simulink model "ProjectFinal"  (R2019a)
settings: Solver=ode45  StartTime=0.6  StopTime=1  MaxStep=1e-7  MinStep=1e-8  RelTol=1e-3
undefined symbols (not defined in the file): sigbuilder_block
libraries: powerlib x55, simulink x10, dspstat3 x2, re_lib x1
(part 1 of 2)
settings Model: Creator=Nabila Tasnim  LastModifiedBy=Nabila Tasnim

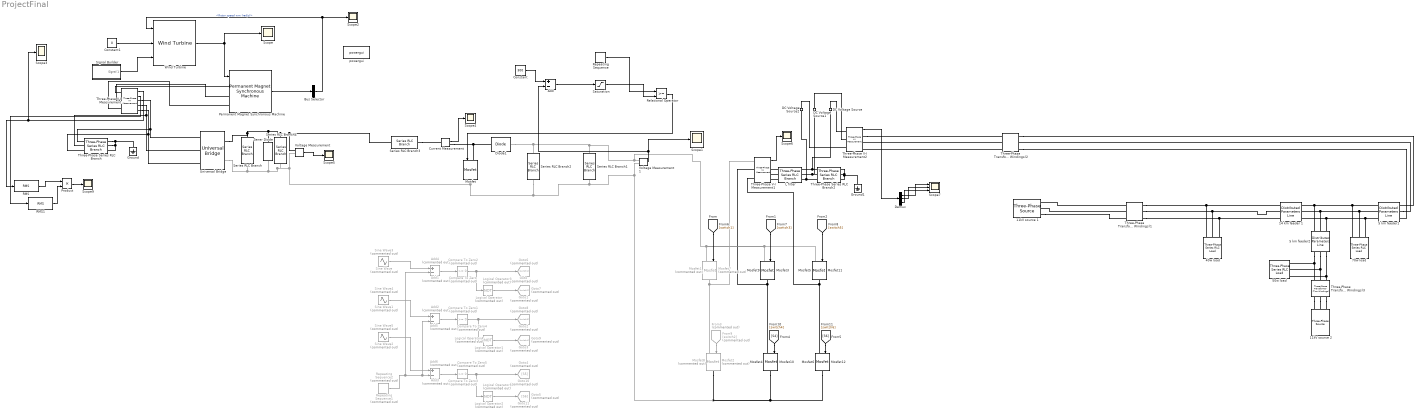
== system ProjectFinal ==
  11kV source 1 : powerlib/Electrical Sources/Three-Phase Source  InternalConnection=Yg  VoltagePhases=off  Voltage=11e3*(1/sqrt(2))  PhaseAngle=0  Voltage_phases=[25e3 25e3 25e3]/sqrt(3)  PhaseAngles_phases=[0 -120 +120]  Frequency=60  NonIdealSource=on  SpecifyImpedance=off  Resistance=0.8929  Inductance=0  ShortCircuitLevel=100e6  BaseVoltage=25e3  XRratio=7  BusType=swing  Pref=0  Qref=0  Prefabc=[10e3, 10e3, 10e3]  Qrefabc=[0, 0, 0]  Qmin=-inf  Qmax=inf
      settings: SourceProductName=Simscape Electrical
  11kV source 2 : powerlib/Electrical Sources/Three-Phase Source  InternalConnection=Yg  VoltagePhases=off  Voltage=11e3*(1/sqrt(2))  PhaseAngle=0  Voltage_phases=[25e3 25e3 25e3]/sqrt(3)  PhaseAngles_phases=[0 -120 +120]  Frequency=60  NonIdealSource=on  SpecifyImpedance=off  Resistance=0.8929  Inductance=0  ShortCircuitLevel=100e6  BaseVoltage=25e3  XRratio=7  BusType=swing  Pref=0  Qref=0  Prefabc=[10e3, 10e3, 10e3]  Qrefabc=[0, 0, 0]  Qmin=-inf  Qmax=inf
      settings: SourceProductName=Simscape Electrical
  14 km feeder 1 : powerlib/Elements/Distributed Parameters Line  Phases=3  Frequency=50  Resistance=[0.01273 0.003864]  Inductance=[0.001 0.001]  Capacitance=[0.001 0.001]  Length=10  x1=[-0.01 -3.68951467134757e-09 40.0386247368383 386.049187884333;-0.0099995 -3.68951467134757e-09 39.9658554684164 386.056728128973;-0.009999 -3.68951467134757e-09 39.8930847799852 386.064254656796;-0.0099985 -3.68951467134757e-09 39.8203126741293 386.071767467533;-0.009998 -3.68951467134757e-09 39.7475391534347 386.079266560918;-0.0099975 -3.68951467134757e-09 39.6747642204872 386.086751936685;-0.009997 -3.68951467134757e-09 39.6019878778729 386.094223594567;-0.0099965 -3.68951467134757e-09 39.5292101281768 386.101681534299;-0.009996 -3.68951467134757e-09 39.456430973985 386.109125755615;-0.0099955 -3.68951467134757e-09 39.3836504178839 386.116556258253;-0.009995 -3.68951467134757e-09 39.3108684624588 386.123973041946;-0.0099945 -3.68951467134757e-09 39.2380851102958 386.131376106433;-0.009994 -3.68951467134757e-09 39.1653003639809 386.13876545145;-0.0099935 -3.68951467134757e-09 39.0925142261009 386.146141076733;-0.009993 -3.68951467134757e-09 39.019726699241 386.153502982023;-0.0099925 -3.68951467134757e-09 38.9469377859875 386.160851167056;-0.009992 -3.68951467134757e-09 38.8741474889275 386.168185631571;-0.0099915 -3.68951467134757e-09 38.8013558106463 386.175506375309;-0.009991 -3.68951467134757e-09 38.7285627537305 386.182813398008;-0.0099905 -3.68951467134757e-09 38.6557683207665 386.19010669941;-0.00999 -3.68951467134757e-09 38.5829725143412 386.197386279255;-0.0099895 -3.68951467134757e-09 38.5101753370404 386.204652137284;-0.009989 -3.68951467134757e-09 38.4373767914507 386.21190427324;-0.0099885 -3.68951467134757e-09 38.3645768801595 386.219142686865;-0.009988 -3.68951467134757e-09 38.2917756057523 386.226367377901;-0.0099875 -3.68951467134757e-09 38.2189729708163 386.233578346092;-0.009987 -3.68951467134757e-09 38.1461689779381 386.240775591181;-0.0099865 -3.68951467134757e-09 38.073363629705 386.247959112913;-0.009986 -3.68951467134757e-09 38.000556928703 386.255128911033;-0.0099855 -3.68951467134757e-09 37.9277488775194 386.262284985286;-0.009985 -3.68951467134757e-09 37.8549394787412 386.269427335417;-0.0099845 -3.68951467134757e-09 37.782128734955 386.276555961174;-0.009984 -3.68951467134757e-09 37.709316648748 386.283670862302;-0.0099835 -3.68951467134757e-09 37.6365032227075 386.290772038548;-0.009983 -3.68951467134757e-09 37.5636884594201 386.297859489661;-0.0099825 -3.68951467134757e-09 37.4908723614733 386.304933215389;-0.009982 -3.68951467134757e-09 37.4180549314543 386.31199321548;-0.0099815 -3.68951467134757e-09 37.3452361719503 386.319039489684;-0.009981 -3.68951467134757e-09 37.2724160855485 386.326072037749;-0.0099805 -3.68951467134757e-09 37.1995946748362 386.333090859427;-0.00998 -3.68951467134757e-09 37.1267719424011 386.340095954468;-0.0099795 -3.68951467134757e-09 37.0539478908302 386.347087322622;-0.009979 -3.68951467134757e-09 36.9811225227113 386.354064963643;-0.0099785 -3.68951467134757e-09 36.9082958406317 386.361028877281;-0.009978 -3.68951467134757e-09 36.8354678471794 386.367979063289;-0.0099775 -3.68951467134757e-09 36.7626385449414 386.37491552142;-0.009977 -3.68951467134757e-09 36.6898079365058 386.381838251428;-0.0099765 -3.68951467134757e-09 36.6169760244603 386.388747253067;-0.009976 -3.68951467134757e-09 36.5441428113925 386.395642526091;-0.0099755 -3.68951467134757e-09 36.4713082998902 386.402524070256;-0.009975 -3.68951467134757e-09 36.3984724925412 386.409391885317;-0.0099745 -3.68951467134757e-09 36.3256353919339 386.416245971029;-0.009974 -3.68951467134757e-09 36.2527970006556 386.42308632715;-0.0099735 -3.68951467134757e-09 36.1799573212945 386.429912953436;-0.009973 -3.68951467134757e-09 36.1071163564389 386.436725849644;-0.0099725 -3.68951467134757e-09 36.0342741086765 386.443525015533;-0.009972 -3.68951467134757e-09 35.9614305805956 386.450310450862;-0.0099715 -3.68951467134757e-09 35.8885857747843 386.457082155388;-0.009971 -3.68951467134757e-09 35.8157396938311 386.463840128872;-0.0099705 -3.68951467134757e-09 35.7428923403239 386.470584371073;-0.00997 ...(+1348205 chars)]  x2=[-0.01 -6.7554586962748e-08 -198.081584719035 -137.663501550197;-0.0099995 -6.75545869719076e-08 -198.055632241504 -137.700836603426;-0.009999 -6.75545869810679e-08 -198.029672726942 -137.738166764065;-0.0099985 -6.75545869902288e-08 -198.003706176272 -137.775492030788;-0.009998 -6.75545869993904e-08 -197.977732590417 -137.812812402268;-0.0099975 -6.75545870085525e-08 -197.951751970298 -137.85012787718;-0.009997 -6.75545870177153e-08 -197.92576431684 -137.887438454197;-0.0099965 -6.75545870268788e-08 -197.899769630966 -137.924744131994;-0.009996 -6.75545870360428e-08 -197.873767913599 -137.962044909245;-0.0099955 -6.75545870452075e-08 -197.847759165662 -137.999340784626;-0.009995 -6.75545870543728e-08 -197.821743388082 -138.036631756811;-0.0099945 -6.75545870635388e-08 -197.79572058178 -138.073917824474;-0.009994 -6.75545870727053e-08 -197.769690747683 -138.111198986292;-0.0099935 -6.75545870818725e-08 -197.743653886715 -138.148475240939;-0.009993 -6.75545870910404e-08 -197.717609999801 -138.185746587092;-0.0099925 -6.75545871002088e-08 -197.691559087866 -138.223013023425;-0.009992 -6.75545871093779e-08 -197.665501151837 -138.260274548615;-0.0099915 -6.75545871185476e-08 -197.639436192638 -138.297531161338;-0.009991 -6.75545871277179e-08 -197.613364211197 -138.33478286027;-0.0099905 -6.75545871368888e-08 -197.587285208439 -138.372029644088;-0.00999 -6.75545871460604e-08 -197.561199185291 -138.409271511468;-0.0099895 -6.75545871552326e-08 -197.535106142679 -138.446508461086;-0.009989 -6.75545871644054e-08 -197.509006081532 -138.483740491621;-0.0099885 -6.75545871735788e-08 -197.482899002776 -138.520967601748;-0.009988 -6.75545871827529e-08 -197.456784907339 -138.558189790146;-0.0099875 -6.75545871919276e-08 -197.430663796149 -138.595407055491;-0.009987 -6.75545872011029e-08 -197.404535670133 -138.632619396462;-0.0099865 -6.75545872102788e-08 -197.378400530221 -138.669826811736;-0.009986 -6.75545872194554e-08 -197.352258377341 -138.707029299992;-0.0099855 -6.75545872286325e-08 -197.326109212421 -138.744226859906;-0.009985 -6.75545872378103e-08 -197.299953036391 -138.781419490159;-0.0099845 -6.75545872469887e-08 -197.27378985018 -138.818607189427;-0.009984 -6.75545872561678e-08 -197.247619654717 -138.855789956391;-0.0099835 -6.75545872653474e-08 -197.221442450933 -138.892967789728;-0.009983 -6.75545872745277e-08 -197.195258239758 -138.930140688119;-0.0099825 -6.75545872837086e-08 -197.169067022122 -138.967308650241;-0.009982 -6.75545872928901e-08 -197.142868798955 -139.004471674775;-0.0099815 -6.75545873020722e-08 -197.116663571188 -139.0416297604;-0.009981 -6.7554587311255e-08 -197.090451339753 -139.078782905796;-0.0099805 -6.75545873204383e-08 -197.064232105581 -139.115931109643;-0.00998 -6.75545873296223e-08 -197.038005869603 -139.15307437062;-0.0099795 -6.75545873388069e-08 -197.011772632752 -139.190212687409;-0.009979 -6.75545873479921e-08 -196.985532395959 -139.22734605869;-0.0099785 -6.7554587357178e-08 -196.959285160156 -139.264474483142;-0.009978 -6.75545873663644e-08 -196.933030926276 -139.301597959448;-0.0099775 -6.75545873755515e-08 -196.906769695253 -139.338716486287;-0.009977 -6.75545873847392e-08 -196.880501468019 -139.375830062342;-0.0099765 -6.75545873939275e-08 -196.854226245507 -139.412938686293;-0.009976 -6.75545874031164e-08 -196.827944028651 -139.450042356823;-0.0099755 -6.75545874123059e-08 -196.801654818385 -139.487141072612;-0.009975 -6.7554587421496e-08 -196.775358615642 -139.524234832342;-0.0099745 -6.75545874306868e-08 -196.749055421358 -139.561323634697;-0.009974 -6.75545874398782e-08 -196.722745236467 -139.598407478357;-0.0099735 -6.75545874490701e-08 -196.696428061904 -139.635486362005;-0.009973 -6.75545874582627e-08 -196.670103898603 -139.672560284324;-0.0099725 -6.75545874674559e-08 -196.6437727475 -139.709629243996;-0.009972 -6.75545874766497e-08 -196.61743460953 -139.746693239705;-0.0099715 -6.75545874858442e-08 -196.59108948563 -139.783752270134;-0.009971 -6.75545874950392e-08 ...(+1336817 chars)]  x3=[-0.01 -1.62478057315764e-06 -221.432025815837 44.6071475712504;-0.0099995 -1.62478057315087e-06 -221.44043013121 44.5654078255042;-0.009999 -1.6247805731441e-06 -221.448826578677 44.5236664963238;-0.0099985 -1.62478057313733e-06 -221.45721515794 44.4819235851916;-0.009998 -1.62478057313055e-06 -221.4655958687 44.440179093591;-0.0099975 -1.62478057312377e-06 -221.47396871066 44.3984330230054;-0.009997 -1.62478057311699e-06 -221.482333683523 44.3566853749181;-0.0099965 -1.62478057311021e-06 -221.49069078699 44.314936150812;-0.009996 -1.62478057310343e-06 -221.499040020766 44.2731853521706;-0.0099955 -1.62478057309664e-06 -221.507381384554 44.2314329804777;-0.009995 -1.62478057308985e-06 -221.515714878057 44.1896790372164;-0.0099945 -1.62478057308305e-06 -221.524040500979 44.1479235238703;-0.009994 -1.62478057307626e-06 -221.532358253024 44.106166441923;-0.0099935 -1.62478057306946e-06 -221.540668133897 44.0644077928585;-0.009993 -1.62478057306266e-06 -221.548970143302 44.02264757816;-0.0099925 -1.62478057305586e-06 -221.557264280945 43.9808857993114;-0.009992 -1.62478057304905e-06 -221.565550546531 43.9391224577969;-0.0099915 -1.62478057304224e-06 -221.573828939765 43.8973575550999;-0.009991 -1.62478057303543e-06 -221.582099460354 43.8555910927045;-0.0099905 -1.62478057302862e-06 -221.590362108003 43.8138230720946;-0.00999 -1.62478057302181e-06 -221.598616882419 43.7720534947546;-0.0099895 -1.62478057301499e-06 -221.606863783308 43.7302823621682;-0.009989 -1.62478057300817e-06 -221.615102810378 43.6885096758196;-0.0099885 -1.62478057300135e-06 -221.623333963336 43.6467354371934;-0.009988 -1.62478057299452e-06 -221.631557241889 43.6049596477733;-0.0099875 -1.62478057298769e-06 -221.639772645745 43.5631823090439;-0.009987 -1.62478057298086e-06 -221.647980174613 43.5214034224895;-0.0099865 -1.62478057297403e-06 -221.6561798282 43.4796229895948;-0.009986 -1.6247805729672e-06 -221.664371606215 43.4378410118439;-0.0099855 -1.62478057296036e-06 -221.672555508368 43.3960574907215;-0.009985 -1.62478057295352e-06 -221.680731534367 43.3542724277123;-0.0099845 -1.62478057294668e-06 -221.688899683923 43.3124858243007;-0.009984 -1.62478057293983e-06 -221.697059956744 43.2706976819716;-0.0099835 -1.62478057293299e-06 -221.70521235254 43.2289080022098;-0.009983 -1.62478057292614e-06 -221.713356871023 43.1871167864999;-0.0099825 -1.62478057291928e-06 -221.721493511903 43.1453240363268;-0.009982 -1.62478057291243e-06 -221.729622274891 43.1035297531756;-0.0099815 -1.62478057290557e-06 -221.737743159697 43.0617339385312;-0.009981 -1.62478057289871e-06 -221.745856166033 43.0199365938785;-0.0099805 -1.62478057289185e-06 -221.753961293612 42.9781377207027;-0.00998 -1.62478057288499e-06 -221.762058542145 42.9363373204891;-0.0099795 -1.62478057287812e-06 -221.770147911344 42.8945353947225;-0.009979 -1.62478057287125e-06 -221.778229400922 42.8527319448885;-0.0099785 -1.62478057286438e-06 -221.786303010592 42.8109269724721;-0.009978 -1.62478057285751e-06 -221.794368740067 42.769120478959;-0.0099775 -1.62478057285063e-06 -221.80242658906 42.7273124658343;-0.009977 -1.62478057284375e-06 -221.810476557286 42.6855029345837;-0.0099765 -1.62478057283687e-06 -221.818518644457 42.6436918866926;-0.009976 -1.62478057282999e-06 -221.826552850289 42.6018793236465;-0.0099755 -1.6247805728231e-06 -221.834579174495 42.5600652469311;-0.009975 -1.62478057281621e-06 -221.842597616792 42.518249658032;-0.0099745 -1.62478057280932e-06 -221.850608176893 42.4764325584352;-0.009974 -1.62478057280243e-06 -221.858610854514 42.4346139496262;-0.0099735 -1.62478057279553e-06 -221.866605649371 42.3927938330908;-0.009973 -1.62478057278863e-06 -221.87459256118 42.3509722103153;-0.0099725 -1.62478057278173e-06 -221.882571589657 42.3091490827852;-0.009972 -1.62478057277483e-06 -221.890542734518 42.2673244519867;-0.0099715 -1.62478057276792e-06 -221.89850599548 42.2254983194058;-0.009971 -1.62478057276102e-06 -221.906461372261 42.1836706865287;-0.0099705 -1.62478057275411e-06 ...(+1344161 chars)]  x4=[-0.01 1.55556818485821e-06 -588.489188137571 -340.386028198852;-0.0099995 1.55556818483735e-06 -588.425016428536 -340.49694974975;-0.009999 1.5555681848165e-06 -588.360823812423 -340.607859202594;-0.0099985 1.55556818479565e-06 -588.29661029151 -340.718756553446;-0.009998 1.5555681847748e-06 -588.23237586808 -340.829641798364;-0.0099975 1.55556818475395e-06 -588.168120544414 -340.940514933409;-0.009997 1.5555681847331e-06 -588.103844322798 -341.05137595464;-0.0099965 1.55556818471226e-06 -588.039547205513 -341.16222485812;-0.009996 1.55556818469141e-06 -587.975229194844 -341.27306163991;-0.0099955 1.55556818467057e-06 -587.910890293077 -341.383886296071;-0.009995 1.55556818464974e-06 -587.846530502497 -341.494698822667;-0.0099945 1.5555681846289e-06 -587.782149825392 -341.605499215759;-0.009994 1.55556818460807e-06 -587.717748264048 -341.716287471411;-0.0099935 1.55556818458723e-06 -587.653325820755 -341.827063585686;-0.009993 1.5555681845664e-06 -587.5888824978 -341.93782755465;-0.0099925 1.55556818454558e-06 -587.524418297474 -342.048579374365;-0.009992 1.55556818452475e-06 -587.459933222068 -342.159319040897;-0.0099915 1.55556818450393e-06 -587.395427273872 -342.270046550312;-0.009991 1.55556818448311e-06 -587.330900455178 -342.380761898675;-0.0099905 1.55556818446229e-06 -587.266352768278 -342.491465082053;-0.00999 1.55556818444147e-06 -587.201784215468 -342.602156096511;-0.0099895 1.55556818442065e-06 -587.13719479904 -342.712834938118;-0.009989 1.55556818439984e-06 -587.072584521289 -342.82350160294;-0.0099885 1.55556818437903e-06 -587.007953384512 -342.934156087046;-0.009988 1.55556818435822e-06 -586.943301391003 -343.044798386504;-0.0099875 1.55556818433741e-06 -586.878628543062 -343.155428497382;-0.009987 1.55556818431661e-06 -586.813934842984 -343.266046415751;-0.0099865 1.5555681842958e-06 -586.749220293071 -343.376652137679;-0.009986 1.555568184275e-06 -586.684484895619 -343.487245659238;-0.0099855 1.5555681842542e-06 -586.61972865293 -343.597826976497;-0.009985 1.55556818423341e-06 -586.554951567304 -343.708396085526;-0.0099845 1.55556818421261e-06 -586.490153641043 -343.818952982399;-0.009984 1.55556818419182e-06 -586.425334876449 -343.929497663187;-0.0099835 1.55556818417103e-06 -586.360495275825 -344.040030123961;-0.009983 1.55556818415024e-06 -586.295634841475 -344.150550360796;-0.0099825 1.55556818412945e-06 -586.230753575704 -344.261058369763;-0.009982 1.55556818410867e-06 -586.165851480817 -344.371554146936;-0.0099815 1.55556818408789e-06 -586.10092855912 -344.48203768839;-0.009981 1.55556818406711e-06 -586.035984812919 -344.592508990198;-0.0099805 1.55556818404633e-06 -585.971020244522 -344.702968048437;-0.00998 1.55556818402555e-06 -585.906034856237 -344.81341485918;-0.0099795 1.55556818400478e-06 -585.841028650374 -344.923849418504;-0.009979 1.55556818398401e-06 -585.776001629241 -345.034271722486;-0.0099785 1.55556818396324e-06 -585.710953795151 -345.144681767201;-0.009978 1.55556818394247e-06 -585.645885150412 -345.255079548727;-0.0099775 1.5555681839217e-06 -585.580795697338 -345.365465063141;-0.009977 1.55556818390094e-06 -585.515685438242 -345.475838306521;-0.0099765 1.55556818388018e-06 -585.450554375436 -345.586199274945;-0.009976 1.55556818385942e-06 -585.385402511234 -345.696547964494;-0.0099755 1.55556818383866e-06 -585.320229847953 -345.806884371245;-0.009975 1.5555681838179e-06 -585.255036387906 -345.917208491278;-0.0099745 1.55556818379715e-06 -585.189822133411 -346.027520320673;-0.009974 1.5555681837764e-06 -585.124587086785 -346.137819855512;-0.0099735 1.55556818375565e-06 -585.059331250346 -346.248107091874;-0.009973 1.5555681837349e-06 -584.994054626411 -346.358382025842;-0.0099725 1.55556818371416e-06 -584.928757217301 -346.468644653497;-0.009972 1.55556818369341e-06 -584.863439025335 -346.578894970922;-0.0099715 1.55556818367267e-06 -584.798100052835 -346.689132974199;-0.009971 1.55556818365193e-06 -584.732740302122 -346.799358659411;-0.0099705 1.5555681836312e-06 -584.667359775517 ...(+1317200 chars)]  x5=0.01  V1=[7.671e-10 1.391e+04 1.391e+04;377 377 377;1.713 0.5014 -1.069]  V2=[7.133e-10 1.392e+04 1.392e+04;377 377 377;1.657 0.5006 -1.07]  I1=[1.903e-12 49.09 49.09;377 377 377;-2.313 0.4756 -1.095]  I2=[4.015e-12 53.69 53.69;377 377 377;1.157 0.5068 -1.064]  nHarmo=1  Measurements=None
      settings: SourceProductName=Simscape Electrical
  40w load : powerlib/Elements/Three-Phase Series RLC Load  LConnTagsString=A|B|C  Configuration=Y (grounded)  NominalVoltage=220e3  Vabc=[1e3 1e3 1e3]  Vabcp=[1e3 1e3 1e3]  NominalFrequency=50  UnbalancedPower=off  ActivePower=40  InductivePower=30  CapacitivePower=30  Pabc=[10e3 9e3 11e3]  QLabc=[100 90 110]  QCabc=[100 90 110]  Pabcp=[10e3 9e3 11e3]  QLabcp=[100 90 110]  QCabcp=[100 90 110]  Measurements=None  LoadType=constant Z
      settings: SourceProductName=Simscape Electrical
  5 km feeder1 : powerlib/Elements/Distributed Parameters Line  Phases=3  Frequency=50  Resistance=[0.01273 0.003864]  Inductance=[0.001 0.001]  Capacitance=[0.001 0.001]  Length=5  x1=[-0.005 -6.75546507364053e-08 192.136346156239 -145.846420420928;-0.0049995 -6.75546507357033e-08 192.163834145296 -145.810200982124;-0.004999 -6.75546507349997e-08 192.191315306661 -145.7739763626;-0.0049985 -6.75546507342944e-08 192.218789639357 -145.737746563643;-0.004998 -6.75546507335875e-08 192.24625714241 -145.70151158654;-0.0049975 -6.75546507328789e-08 192.273717814842 -145.665271432578;-0.004997 -6.75546507321687e-08 192.301171655679 -145.629026103045;-0.0049965 -6.75546507314569e-08 192.328618663944 -145.592775599229;-0.004996 -6.75546507307434e-08 192.356058838662 -145.556519922418;-0.0049955 -6.75546507300283e-08 192.383492178859 -145.5202590739;-0.004995 -6.75546507293116e-08 192.41091868356 -145.483993054964;-0.0049945 -6.75546507285932e-08 192.43833835179 -145.447721866897;-0.004994 -6.75546507278732e-08 192.465751182575 -145.411445510989;-0.0049935 -6.75546507271516e-08 192.493157174941 -145.375163988529;-0.004993 -6.75546507264283e-08 192.520556327914 -145.338877300805;-0.0049925 -6.75546507257034e-08 192.547948640522 -145.302585449108;-0.004992 -6.75546507249768e-08 192.575334111789 -145.266288434726;-0.0049915 -6.75546507242486e-08 192.602712740745 -145.229986258949;-0.004991 -6.75546507235188e-08 192.630084526415 -145.193678923067;-0.0049905 -6.75546507227874e-08 192.657449467827 -145.15736642837;-0.00499 -6.75546507220543e-08 192.684807564009 -145.121048776148;-0.0049895 -6.75546507213195e-08 192.712158813989 -145.084725967692;-0.004989 -6.75546507205832e-08 192.739503216795 -145.048398004292;-0.0049885 -6.75546507198452e-08 192.766840771455 -145.012064887238;-0.004988 -6.75546507191056e-08 192.794171476999 -144.975726617823;-0.0049875 -6.75546507183643e-08 192.821495332455 -144.939383197337;-0.004987 -6.75546507176214e-08 192.848812336852 -144.903034627071;-0.0049865 -6.75546507168769e-08 192.876122489219 -144.866680908316;-0.004986 -6.75546507161307e-08 192.903425788587 -144.830322042365;-0.0049855 -6.75546507153829e-08 192.930722233985 -144.79395803051;-0.004985 -6.75546507146335e-08 192.958011824444 -144.757588874042;-0.0049845 -6.75546507138824e-08 192.985294558993 -144.721214574253;-0.004984 -6.75546507131297e-08 193.012570436664 -144.684835132436;-0.0049835 -6.75546507123753e-08 193.039839456487 -144.648450549884;-0.004983 -6.75546507116194e-08 193.067101617493 -144.612060827888;-0.0049825 -6.75546507108617e-08 193.094356918714 -144.575665967744;-0.004982 -6.75546507101025e-08 193.121605359181 -144.539265970742;-0.0049815 -6.75546507093416e-08 193.148846937927 -144.502860838177;-0.004981 -6.75546507085791e-08 193.176081653982 -144.466450571343;-0.0049805 -6.75546507078149e-08 193.203309506381 -144.430035171532;-0.00498 -6.75546507070492e-08 193.230530494154 -144.393614640038;-0.0049795 -6.75546507062817e-08 193.257744616336 -144.357188978157;-0.004979 -6.75546507055127e-08 193.284951871958 -144.320758187182;-0.0049785 -6.7554650704742e-08 193.312152260055 -144.284322268407;-0.004978 -6.75546507039697e-08 193.33934577966 -144.247881223126;-0.0049775 -6.75546507031957e-08 193.366532429807 -144.211435052636;-0.004977 -6.75546507024201e-08 193.393712209529 -144.17498375823;-0.0049765 -6.75546507016429e-08 193.420885117862 -144.138527341204;-0.004976 -6.7554650700864e-08 193.448051153839 -144.102065802854;-0.0049755 -6.75546507000835e-08 193.475210316495 -144.065599144473;-0.004975 -6.75546506993014e-08 193.502362604866 -144.02912736736;-0.0049745 -6.75546506985176e-08 193.529508017987 -143.992650472808;-0.004974 -6.75546506977322e-08 193.556646554892 -143.956168462115;-0.0049735 -6.75546506969452e-08 193.583778214619 -143.919681336576;-0.004973 -6.75546506961565e-08 193.610902996202 -143.883189097488;-0.0049725 -6.75546506953662e-08 193.638020898679 -143.846691746147;-0.004972 -6.75546506945743e-08 193.665131921085 -143.810189283851;-0.0049715 -6.75546506937807e-08 193.692236062458 -143.773681711895;-0.004971 -6.75546506929855e-08 193.719333321834 -143.737169031579;-0.0049705 -6.75546506921887e-08 ...(+660401 chars)]  x2=[-0.005 -9.94910147324311e-08 -660.902247034562 406.799019620361;-0.0049995 -9.94910147228076e-08 -660.97891510168 406.674435255556;-0.004999 -9.94910147131766e-08 -661.055559683838 406.549836441373;-0.0049985 -9.94910147035381e-08 -661.132180778311 406.425223182241;-0.004998 -9.94910146938921e-08 -661.208778382377 406.300595482587;-0.0049975 -9.94910146842386e-08 -661.285352493314 406.175953346839;-0.004997 -9.94910146745777e-08 -661.361903108402 406.051296779425;-0.0049965 -9.94910146649092e-08 -661.43843022492 405.926625784775;-0.004996 -9.94910146552333e-08 -661.514933840151 405.801940367318;-0.0049955 -9.94910146455498e-08 -661.591413951375 405.677240531485;-0.004995 -9.94910146358589e-08 -661.667870555875 405.552526281706;-0.0049945 -9.94910146261605e-08 -661.744303650935 405.427797622411;-0.004994 -9.94910146164546e-08 -661.820713233838 405.303054558034;-0.0049935 -9.94910146067412e-08 -661.897099301871 405.178297093006;-0.004993 -9.94910145970204e-08 -661.973461852319 405.05352523176;-0.0049925 -9.9491014587292e-08 -662.049800882468 404.928738978729;-0.004992 -9.94910145775562e-08 -662.126116389607 404.803938338346;-0.0049915 -9.94910145678128e-08 -662.202408371024 404.679123315047;-0.004991 -9.9491014558062e-08 -662.278676824008 404.554293913265;-0.0049905 -9.94910145483037e-08 -662.354921745849 404.429450137437;-0.00499 -9.9491014538538e-08 -662.431143133839 404.304591991997;-0.0049895 -9.94910145287647e-08 -662.507340985268 404.179719481382;-0.004989 -9.9491014518984e-08 -662.583515297431 404.054832610029;-0.0049885 -9.94910145091957e-08 -662.659666067619 403.929931382376;-0.004988 -9.94910144994e-08 -662.735793293128 403.805015802859;-0.0049875 -9.94910144895968e-08 -662.811896971253 403.680085875917;-0.004987 -9.94910144797862e-08 -662.88797709929 403.55514160599;-0.0049865 -9.9491014469968e-08 -662.964033674535 403.430182997516;-0.004986 -9.94910144601424e-08 -663.040066694286 403.305210054936;-0.0049855 -9.94910144503092e-08 -663.116076155842 403.180222782689;-0.004985 -9.94910144404686e-08 -663.192062056502 403.055221185217;-0.0049845 -9.94910144306206e-08 -663.268024393566 402.930205266961;-0.004984 -9.9491014420765e-08 -663.343963164336 402.805175032362;-0.0049835 -9.94910144109019e-08 -663.419878366112 402.680130485864;-0.004983 -9.94910144010314e-08 -663.495769996199 402.555071631909;-0.0049825 -9.94910143911534e-08 -663.571638051898 402.42999847494;-0.004982 -9.94910143812679e-08 -663.647482530515 402.304911019402;-0.0049815 -9.9491014371375e-08 -663.723303429355 402.179809269739;-0.004981 -9.94910143614745e-08 -663.799100745724 402.054693230395;-0.0049805 -9.94910143515666e-08 -663.874874476929 401.929562905817;-0.00498 -9.94910143416512e-08 -663.950624620277 401.80441830045;-0.0049795 -9.94910143317284e-08 -664.026351173078 401.679259418741;-0.004979 -9.9491014321798e-08 -664.102054132639 401.554086265136;-0.0049785 -9.94910143118602e-08 -664.177733496273 401.428898844084;-0.004978 -9.94910143019149e-08 -664.253389261289 401.303697160031;-0.0049775 -9.94910142919621e-08 -664.329021424999 401.178481217428;-0.004977 -9.94910142820019e-08 -664.404629984718 401.053251020722;-0.0049765 -9.94910142720342e-08 -664.480214937757 400.928006574362;-0.004976 -9.9491014262059e-08 -664.555776281431 400.8027478828;-0.0049755 -9.94910142520763e-08 -664.631314013056 400.677474950486;-0.004975 -9.94910142420861e-08 -664.706828129948 400.55218778187;-0.0049745 -9.94910142320885e-08 -664.782318629424 400.426886381405;-0.004974 -9.94910142220834e-08 -664.857785508801 400.301570753541;-0.0049735 -9.94910142120709e-08 -664.933228765398 400.176240902733;-0.004973 -9.94910142020508e-08 -665.008648396535 400.050896833432;-0.0049725 -9.94910141920233e-08 -665.084044399532 399.925538550092;-0.004972 -9.94910141819883e-08 -665.159416771709 399.800166057168;-0.0049715 -9.94910141719459e-08 -665.23476551039 399.674779359113;-0.004971 -9.94910141618959e-08 -665.310090612896 399.549378460384;-0.0049705 -9.94910141518386e-08 ...(+673975 chars)]  x3=[-0.005 -1.70370472781793e-06 544.635993719938 478.008313803511;-0.0049995 -1.70370472784795e-06 544.545881600436 478.110966777152;-0.004999 -1.70370472787796e-06 544.455750132906 478.213602763237;-0.0049985 -1.70370472790797e-06 544.365599320549 478.316221758116;-0.004998 -1.70370472793798e-06 544.275429166569 478.418823758144;-0.0049975 -1.70370472796798e-06 544.18523967417 478.521408759677;-0.004997 -1.70370472799798e-06 544.095030846556 478.623976759068;-0.0049965 -1.70370472802797e-06 544.004802686933 478.726527752673;-0.004996 -1.70370472805796e-06 543.914555198505 478.82906173685;-0.0049955 -1.70370472808795e-06 543.82428838448 478.931578707954;-0.004995 -1.70370472811793e-06 543.734002248065 479.034078662344;-0.0049945 -1.7037047281479e-06 543.643696792468 479.136561596377;-0.004994 -1.70370472817787e-06 543.553372020898 479.239027506412;-0.0049935 -1.70370472820784e-06 543.463027936563 479.341476388808;-0.004993 -1.7037047282378e-06 543.372664542674 479.443908239926;-0.0049925 -1.70370472826776e-06 543.282281842441 479.546323056126;-0.004992 -1.70370472829771e-06 543.191879839076 479.648720833769;-0.0049915 -1.70370472832766e-06 543.101458535791 479.751101569216;-0.004991 -1.7037047283576e-06 543.011017935798 479.853465258831;-0.0049905 -1.70370472838754e-06 542.920558042311 479.955811898976;-0.00499 -1.70370472841748e-06 542.830078858545 480.058141486014;-0.0049895 -1.70370472844741e-06 542.739580387713 480.160454016311;-0.004989 -1.70370472847733e-06 542.649062633031 480.26274948623;-0.0049885 -1.70370472850726e-06 542.558525597715 480.365027892137;-0.004988 -1.70370472853717e-06 542.467969284983 480.467289230398;-0.0049875 -1.70370472856709e-06 542.377393698051 480.569533497379;-0.004987 -1.70370472859699e-06 542.286798840139 480.671760689448;-0.0049865 -1.7037047286269e-06 542.196184714464 480.773970802973;-0.004986 -1.7037047286568e-06 542.105551324247 480.876163834322;-0.0049855 -1.70370472868669e-06 542.014898672707 480.978339779864;-0.004985 -1.70370472871658e-06 541.924226763066 481.080498635969;-0.0049845 -1.70370472874647e-06 541.833535598545 481.182640399007;-0.004984 -1.70370472877635e-06 541.742825182367 481.284765065348;-0.0049835 -1.70370472880622e-06 541.652095517754 481.386872631365;-0.004983 -1.7037047288361e-06 541.56134660793 481.488963093429;-0.0049825 -1.70370472886596e-06 541.47057845612 481.591036447912;-0.004982 -1.70370472889583e-06 541.379791065549 481.693092691189;-0.0049815 -1.70370472892568e-06 541.288984439442 481.795131819633;-0.004981 -1.70370472895554e-06 541.198158581025 481.897153829619;-0.0049805 -1.70370472898539e-06 541.107313493527 481.999158717521;-0.00498 -1.70370472901523e-06 541.016449180174 482.101146479716;-0.0049795 -1.70370472904507e-06 540.925565644195 482.203117112579;-0.004979 -1.70370472907491e-06 540.834662888819 482.305070612488;-0.0049785 -1.70370472910474e-06 540.743740917276 482.407006975821;-0.004978 -1.70370472913457e-06 540.652799732797 482.508926198954;-0.0049775 -1.70370472916439e-06 540.561839338613 482.610828278268;-0.004977 -1.70370472919421e-06 540.470859737955 482.71271321014;-0.0049765 -1.70370472922402e-06 540.379860934057 482.814580990953;-0.004976 -1.70370472925383e-06 540.288842930151 482.916431617085;-0.0049755 -1.70370472928363e-06 540.197805729471 483.018265084919;-0.004975 -1.70370472931343e-06 540.106749335252 483.120081390835;-0.0049745 -1.70370472934323e-06 540.01567375073 483.221880531217;-0.004974 -1.70370472937302e-06 539.924578979139 483.323662502447;-0.0049735 -1.7037047294028e-06 539.833465023718 483.425427300909;-0.004973 -1.70370472943259e-06 539.742331887703 483.527174922987;-0.0049725 -1.70370472946236e-06 539.651179574332 483.628905365067;-0.004972 -1.70370472949214e-06 539.560008086843 483.730618623533;-0.0049715 -1.7037047295219e-06 539.468817428477 483.832314694771;-0.004971 -1.70370472955167e-06 539.377607602474 483.933993575169;-0.0049705 -1.70370472958143e-06 539.286378612073 484.035655261114;-0.00497 ...(+662390 chars)]  x4=[-0.005 1.53906017075614e-06 -630.170887454766 387.883231371545;-0.0049995 1.5390601707354e-06 -630.243990525774 387.764440067559;-0.004999 1.53906017071466e-06 -630.317071203849 387.645634986079;-0.0049985 1.53906017069392e-06 -630.390129486396 387.526816131327;-0.004998 1.53906017067319e-06 -630.46316537082 387.407983507523;-0.0049975 1.53906017065247e-06 -630.536178854523 387.289137118892;-0.004997 1.53906017063175e-06 -630.609169934914 387.170276969654;-0.0049965 1.53906017061103e-06 -630.682138609397 387.051403064033;-0.004996 1.53906017059032e-06 -630.755084875381 386.932515406253;-0.0049955 1.53906017056962e-06 -630.828008730273 386.813614000538;-0.004995 1.53906017054893e-06 -630.900910171483 386.694698851113;-0.0049945 1.53906017052823e-06 -630.973789196421 386.575769962202;-0.004994 1.53906017050755e-06 -631.046645802497 386.456827338032;-0.0049935 1.53906017048687e-06 -631.119479987122 386.337870982827;-0.004993 1.53906017046619e-06 -631.192291747708 386.218900900817;-0.0049925 1.53906017044552e-06 -631.265081081669 386.099917096226;-0.004992 1.53906017042486e-06 -631.337847986419 385.980919573283;-0.0049915 1.5390601704042e-06 -631.41059245937 385.861908336215;-0.004991 1.53906017038355e-06 -631.483314497941 385.742883389252;-0.0049905 1.5390601703629e-06 -631.556014099545 385.623844736622;-0.00499 1.53906017034226e-06 -631.628691261601 385.504792382555;-0.0049895 1.53906017032163e-06 -631.701345981525 385.38572633128;-0.004989 1.539060170301e-06 -631.773978256737 385.266646587029;-0.0049885 1.53906017028037e-06 -631.846588084656 385.147553154032;-0.004988 1.53906017025975e-06 -631.919175462702 385.028446036521;-0.0049875 1.53906017023914e-06 -631.991740388295 384.909325238728;-0.004987 1.53906017021853e-06 -632.064282858859 384.790190764884;-0.0049865 1.53906017019793e-06 -632.136802871814 384.671042619224;-0.004986 1.53906017017734e-06 -632.209300424585 384.551880805979;-0.0049855 1.53906017015674e-06 -632.281775514595 384.432705329386;-0.004985 1.53906017013616e-06 -632.35422813927 384.313516193676;-0.0049845 1.53906017011558e-06 -632.426658296035 384.194313403087;-0.004984 1.53906017009501e-06 -632.499065982317 384.075096961852;-0.0049835 1.53906017007444e-06 -632.571451195543 383.955866874208;-0.004983 1.53906017005387e-06 -632.643813933141 383.83662314439;-0.0049825 1.53906017003332e-06 -632.71615419254 383.717365776637;-0.004982 1.53906017001276e-06 -632.78847197117 383.598094775185;-0.0049815 1.53906016999222e-06 -632.860767266461 383.478810144271;-0.004981 1.53906016997168e-06 -632.933040075844 383.359511888135;-0.0049805 1.53906016995114e-06 -633.005290396753 383.240200011014;-0.00498 1.53906016993061e-06 -633.077518226619 383.120874517149;-0.0049795 1.53906016991009e-06 -633.149723562876 383.001535410778;-0.004979 1.53906016988957e-06 -633.221906402959 382.882182696142;-0.0049785 1.53906016986906e-06 -633.294066744303 382.762816377482;-0.004978 1.53906016984855e-06 -633.366204584344 382.643436459038;-0.0049775 1.53906016982805e-06 -633.43831992052 382.524042945053;-0.004977 1.53906016980755e-06 -633.510412750267 382.404635839769;-0.0049765 1.53906016978706e-06 -633.582483071024 382.285215147427;-0.004976 1.53906016976658e-06 -633.654530880231 382.165780872272;-0.0049755 1.5390601697461e-06 -633.726556175328 382.046333018546;-0.004975 1.53906016972563e-06 -633.798558953756 381.926871590495;-0.0049745 1.53906016970516e-06 -633.870539212955 381.807396592362;-0.004974 1.5390601696847e-06 -633.94249695037 381.687908028392;-0.0049735 1.53906016966424e-06 -634.014432163442 381.568405902831;-0.004973 1.53906016964379e-06 -634.086344849617 381.448890219925;-0.0049725 1.53906016962334e-06 -634.158235006339 381.32936098392;-0.004972 1.5390601696029e-06 -634.230102631054 381.209818199063;-0.0049715 1.53906016958247e-06 -634.301947721208 381.090261869602;-0.004971 1.53906016956204e-06 -634.373770274248 380.970691999785;-0.0049705 1.53906016954162e-06 -634.445570287623 380.85110859386;-0.00497 1.5390601695212e-06 ...(+663970 chars)]  x5=0.005  V1=[7.133e-10 1.392e+04 1.392e+04;377 377 377;1.676 0.5123 -1.059]  V2=[7.264e-10 1.392e+04 1.392e+04;377 377 377;1.669 0.5123 -1.059]  I1=[1.636e-12 51.4 51.4;377 377 377;0.6309 0.5058 -1.065]  I2=[1.868e-12 51.4 51.4;377 377 377;2.957 0.5123 -1.059]  nHarmo=1  Measurements=None
      settings: SourceProductName=Simscape Electrical
  5 km feeder2 : powerlib/Elements/Distributed Parameters Line  Phases=3  Frequency=50  Resistance=[0.01273 0.003864]  Inductance=[0.001 0.001]  Capacitance=[0.001 0.001]  Length=2  x1=[-0.0020005 -6.75546209442471e-08 10.1522821596812 -241.007230245948;-0.002 -6.75546209360972e-08 10.1068531869519 -241.009139624477;-0.0019995 -6.75546209279468e-08 10.0614238551202 -241.011040439812;-0.001999 -6.75546209197958e-08 10.0159941658004 -241.012932691886;-0.0019985 -6.75546209116442e-08 9.97056412060647 -241.014816380633;-0.001998 -6.75546209034921e-08 9.92513372115269 -241.016691505983;-0.0019975 -6.75546208953393e-08 9.8797029690532 -241.018558067873;-0.001997 -6.7554620887186e-08 9.83427186592217 -241.020416066233;-0.0019965 -6.75546208790322e-08 9.78884041337381 -241.022265501;-0.001996 -6.75546208708777e-08 9.74340861302228 -241.024106372107;-0.0019955 -6.75546208627227e-08 9.69797646648193 -241.025938679489;-0.001995 -6.75546208545671e-08 9.6525439753668 -241.02776242308;-0.0019945 -6.75546208464109e-08 9.60711114129124 -241.029577602816;-0.001994 -6.75546208382542e-08 9.56167796586949 -241.031384218633;-0.0019935 -6.75546208300968e-08 9.51624445071581 -241.033182270465;-0.001993 -6.75546208219389e-08 9.47081059744449 -241.03497175825;-0.0019925 -6.75546208137805e-08 9.42537640766985 -241.036752681924;-0.001992 -6.75546208056214e-08 9.37994188300617 -241.038525041423;-0.0019915 -6.75546207974618e-08 9.33450702506772 -241.040288836684;-0.001991 -6.75546207893016e-08 9.28907183546886 -241.042044067645;-0.0019905 -6.75546207811409e-08 9.24363631582391 -241.043790734244;-0.00199 -6.75546207729796e-08 9.19820046774724 -241.045528836418;-0.0019895 -6.75546207648177e-08 9.15276429285323 -241.047258374105;-0.001989 -6.75546207566552e-08 9.10732779275631 -241.048979347245;-0.0019885 -6.75546207484922e-08 9.06189096907071 -241.050691755775;-0.001988 -6.75546207403286e-08 9.01645382341091 -241.052395599636;-0.0019875 -6.75546207321644e-08 8.97101635739131 -241.054090878766;-0.001987 -6.75546207239996e-08 8.92557857262634 -241.055777593106;-0.0019865 -6.75546207158343e-08 8.88014047073042 -241.057455742595;-0.001986 -6.75546207076684e-08 8.83470205331798 -241.059125327174;-0.0019855 -6.7554620699502e-08 8.78926332200355 -241.060786346784;-0.001985 -6.75546206913349e-08 8.74382427840151 -241.062438801364;-0.0019845 -6.75546206831673e-08 8.69838492412635 -241.064082690858;-0.001984 -6.75546206749992e-08 8.65294526079255 -241.065718015206;-0.0019835 -6.75546206668305e-08 8.60750529001463 -241.06734477435;-0.001983 -6.75546206586612e-08 8.56206501340709 -241.068962968233;-0.0019825 -6.75546206504913e-08 8.51662443258448 -241.070572596797;-0.001982 -6.75546206423209e-08 8.47118354916127 -241.072173659984;-0.0019815 -6.75546206341499e-08 8.42574236475202 -241.073766157738;-0.001981 -6.75546206259783e-08 8.38030088097132 -241.075350090003;-0.0019805 -6.75546206178062e-08 8.33485909943371 -241.076925456722;-0.00198 -6.75546206096335e-08 8.28941702175374 -241.078492257838;-0.0019795 -6.75546206014602e-08 8.243974649546 -241.080050493297;-0.001979 -6.75546205932864e-08 8.19853198442515 -241.081600163043;-0.0019785 -6.7554620585112e-08 8.15308902800569 -241.083141267021;-0.001978 -6.75546205769371e-08 8.10764578190227 -241.084673805177;-0.0019775 -6.75546205687616e-08 8.06220224772954 -241.086197777454;-0.001977 -6.75546205605855e-08 8.01675842710215 -241.087713183801;-0.0019765 -6.75546205524088e-08 7.97131432163468 -241.089220024162;-0.001976 -6.75546205442316e-08 7.92586993294187 -241.090718298485;-0.0019755 -6.75546205360539e-08 7.88042526263829 -241.092208006715;-0.001975 -6.75546205278755e-08 7.83498031233868 -241.0936891488;-0.0019745 -6.75546205196966e-08 7.78953508365772 -241.095161724688;-0.001974 -6.75546205115172e-08 7.74408957821008 -241.096625734326;-0.0019735 -6.75546205033372e-08 7.69864379761049 -241.098081177662;-0.001973 -6.75546204951566e-08 7.65319774347362 -241.099528054645;-0.0019725 -6.75546204869754e-08 7.6077514174143 -241.100966365222;-0.001972 -6.75546204787937e-08 7.56230482104713 -241.102396109343;-0.0019715 -6.75546204706115e-08 7.51685795598694 -241.103817286958;-0.001971 -6.75546204624287e-08 ...(+268058 chars)]  x2=[-0.0020005 -6.75532475471173e-08 311.802978663309 -615.872282161771;-0.002 -6.75532475104943e-08 311.686883934496 -615.931044697103;-0.0019995 -6.75532474738676e-08 311.570778131268 -615.98978534805;-0.001999 -6.75532474372371e-08 311.45466125775 -616.048504112525;-0.0019985 -6.7553247400603e-08 311.33853331807 -616.107200988443;-0.001998 -6.75532473639651e-08 311.222394316352 -616.165875973717;-0.0019975 -6.75532473273235e-08 311.106244256723 -616.224529066262;-0.001997 -6.75532472906783e-08 310.990083143311 -616.283160263995;-0.0019965 -6.75532472540293e-08 310.873910980241 -616.341769564833;-0.001996 -6.75532472173766e-08 310.757727771643 -616.400356966692;-0.0019955 -6.75532471807202e-08 310.641533521643 -616.458922467493;-0.001995 -6.75532471440601e-08 310.525328234371 -616.517466065152;-0.0019945 -6.75532471073963e-08 310.409111913956 -616.575987757592;-0.001994 -6.75532470707289e-08 310.292884564525 -616.634487542731;-0.0019935 -6.75532470340577e-08 310.17664619021 -616.692965418492;-0.001993 -6.75532469973828e-08 310.06039679514 -616.751421382797;-0.0019925 -6.75532469607042e-08 309.944136383446 -616.809855433569;-0.001992 -6.7553246924022e-08 309.827864959259 -616.868267568731;-0.0019915 -6.7553246887336e-08 309.711582526708 -616.926657786209;-0.001991 -6.75532468506464e-08 309.595289089927 -616.985026083927;-0.0019905 -6.75532468139531e-08 309.478984653047 -617.043372459813;-0.00199 -6.7553246777256e-08 309.362669220201 -617.101696911792;-0.0019895 -6.75532467405553e-08 309.246342795521 -617.159999437792;-0.001989 -6.75532467038509e-08 309.13000538314 -617.218280035742;-0.0019885 -6.75532466671429e-08 309.013656987192 -617.276538703572;-0.001988 -6.75532466304311e-08 308.897297611811 -617.334775439211;-0.0019875 -6.75532465937157e-08 308.780927261131 -617.392990240589;-0.001987 -6.75532465569965e-08 308.664545939287 -617.45118310564;-0.0019865 -6.75532465202738e-08 308.548153650414 -617.509354032294;-0.001986 -6.75532464835473e-08 308.431750398648 -617.567503018485;-0.0019855 -6.75532464468171e-08 308.315336188123 -617.625630062147;-0.001985 -6.75532464100833e-08 308.198911022978 -617.683735161216;-0.0019845 -6.75532463733458e-08 308.082474907347 -617.741818313625;-0.001984 -6.75532463366046e-08 307.966027845369 -617.799879517312;-0.0019835 -6.75532462998598e-08 307.849569841181 -617.857918770214;-0.001983 -6.75532462631113e-08 307.73310089892 -617.915936070268;-0.0019825 -6.75532462263591e-08 307.616621022725 -617.973931415413;-0.001982 -6.75532461896033e-08 307.500130216734 -618.031904803588;-0.0019815 -6.75532461528438e-08 307.383628485087 -618.089856232734;-0.001981 -6.75532461160806e-08 307.267115831922 -618.147785700792;-0.0019805 -6.75532460793137e-08 307.15059226138 -618.205693205703;-0.00198 -6.75532460425433e-08 307.034057777601 -618.26357874541;-0.0019795 -6.75532460057691e-08 306.917512384724 -618.321442317855;-0.001979 -6.75532459689913e-08 306.800956086892 -618.379283920984;-0.0019785 -6.75532459322098e-08 306.684388888245 -618.437103552741;-0.001978 -6.75532458954247e-08 306.567810792925 -618.494901211072;-0.0019775 -6.75532458586359e-08 306.451221805074 -618.552676893923;-0.001977 -6.75532458218434e-08 306.334621928835 -618.610430599241;-0.0019765 -6.75532457850474e-08 306.218011168351 -618.668162324974;-0.001976 -6.75532457482476e-08 306.101389527764 -618.725872069071;-0.0019755 -6.75532457114442e-08 305.984757011219 -618.783559829482;-0.001975 -6.75532456746372e-08 305.868113622859 -618.841225604156;-0.0019745 -6.75532456378265e-08 305.751459366829 -618.898869391046;-0.001974 -6.75532456010122e-08 305.634794247273 -618.956491188102;-0.0019735 -6.75532455641942e-08 305.518118268338 -619.014090993278;-0.001973 -6.75532455273726e-08 305.401431434167 -619.071668804527;-0.0019725 -6.75532454905473e-08 305.284733748908 -619.129224619803;-0.001972 -6.75532454537184e-08 305.168025216707 -619.186758437061;-0.0019715 -6.75532454168858e-08 305.05130584171 -619.244270254258;-0.001971 -6.75532453800497e-08 ...(+265817 chars)]  x3=[-0.0020005 -6.69760107329267e-08 657.185794045103 186.397696218254;-0.002 -6.69760107662817e-08 657.220917507785 186.273816303822;-0.0019995 -6.6976010799633e-08 657.25601761903 186.149929770974;-0.001999 -6.69760108329805e-08 657.29109437759 186.026036624112;-0.0019985 -6.69760108663243e-08 657.326147782219 185.902136867637;-0.001998 -6.69760108996643e-08 657.361177831671 185.778230505953;-0.0019975 -6.69760109330005e-08 657.396184524703 185.654317543461;-0.001997 -6.6976010966333e-08 657.431167860069 185.530397984565;-0.0019965 -6.69760109996617e-08 657.466127836528 185.406471833666;-0.001996 -6.69760110329867e-08 657.501064452836 185.282539095169;-0.0019955 -6.69760110663079e-08 657.535977707753 185.158599773476;-0.001995 -6.69760110996253e-08 657.570867600038 185.034653872992;-0.0019945 -6.6976011132939e-08 657.605734128452 184.91070139812;-0.001994 -6.69760111662489e-08 657.640577291756 184.786742353265;-0.0019935 -6.6976011199555e-08 657.675397088711 184.66277674283;-0.001993 -6.69760112328574e-08 657.71019351808 184.53880457122;-0.0019925 -6.69760112661559e-08 657.744966578628 184.41482584284;-0.001992 -6.69760112994507e-08 657.779716269118 184.290840562096;-0.0019915 -6.69760113327418e-08 657.814442588316 184.166848733392;-0.001991 -6.6976011366029e-08 657.849145534989 184.042850361133;-0.0019905 -6.69760113993125e-08 657.883825107902 183.918845449726;-0.00199 -6.69760114325922e-08 657.918481305825 183.794834003577;-0.0019895 -6.69760114658681e-08 657.953114127525 183.670816027091;-0.001989 -6.69760114991403e-08 657.987723571772 183.546791524676;-0.0019885 -6.69760115324086e-08 658.022309637336 183.422760500737;-0.001988 -6.69760115656732e-08 658.056872322989 183.298722959682;-0.0019875 -6.6976011598934e-08 658.091411627503 183.174678905918;-0.001987 -6.6976011632191e-08 658.125927549649 183.050628343852;-0.0019865 -6.69760116654442e-08 658.160420088203 182.926571277892;-0.001986 -6.69760116986936e-08 658.194889241938 182.802507712445;-0.0019855 -6.69760117319393e-08 658.229335009629 182.678437651921;-0.001985 -6.69760117651811e-08 658.263757390054 182.554361100726;-0.0019845 -6.69760117984192e-08 658.298156381987 182.430278063269;-0.001984 -6.69760118316534e-08 658.332531984209 182.30618854396;-0.0019835 -6.69760118648839e-08 658.366884195496 182.182092547207;-0.001983 -6.69760118981106e-08 658.40121301463 182.057990077419;-0.0019825 -6.69760119313335e-08 658.435518440389 181.933881139006;-0.001982 -6.69760119645526e-08 658.469800471555 181.809765736378;-0.0019815 -6.69760119977678e-08 658.504059106909 181.685643873944;-0.001981 -6.69760120309793e-08 658.538294345236 181.561515556114;-0.0019805 -6.6976012064187e-08 658.572506185317 181.437380787299;-0.00198 -6.69760120973909e-08 658.606694625939 181.31323957191;-0.0019795 -6.6976012130591e-08 658.640859665885 181.189091914356;-0.001979 -6.69760121637872e-08 658.675001303943 181.06493781905;-0.0019785 -6.69760121969797e-08 658.709119538898 180.940777290403;-0.001978 -6.69760122301684e-08 658.743214369539 180.816610332825;-0.0019775 -6.69760122633532e-08 658.777285794655 180.692436950729;-0.001977 -6.69760122965343e-08 658.811333813034 180.568257148527;-0.0019765 -6.69760123297115e-08 658.845358423467 180.444070930631;-0.001976 -6.69760123628849e-08 658.879359624745 180.319878301453;-0.0019755 -6.69760123960545e-08 658.913337415661 180.195679265406;-0.001975 -6.69760124292203e-08 658.947291795006 180.071473826903;-0.0019745 -6.69760124623823e-08 658.981222761574 179.947261990357;-0.001974 -6.69760124955405e-08 659.01513031416 179.82304376018;-0.0019735 -6.69760125286948e-08 659.04901445156 179.698819140788;-0.001973 -6.69760125618454e-08 659.082875172568 179.574588136593;-0.0019725 -6.69760125949921e-08 659.116712475982 179.450350752009;-0.001972 -6.6976012628135e-08 659.1505263606 179.326106991452;-0.0019715 -6.6976012661274e-08 659.18431682522 179.201856859334;-0.001971 -6.69760126944093e-08 659.218083868642 179.077600360071;-0.0019705 -6.69760127275407e-08 ...(+262799 chars)]  x4=[-0.0020005 -6.73512603926724e-08 -6.66182593722424 -900.385123651781;-0.002 -6.7351260317237e-08 -6.83154441526199 -900.383851931582;-0.0019995 -6.73512602418021e-08 -7.00126265057097 -900.382548220226;-0.001999 -6.73512601663676e-08 -7.17098063712102 -900.38121251776;-0.0019985 -6.73512600909335e-08 -7.34069836888199 -900.379844824232;-0.001998 -6.73512600155e-08 -7.51041583982372 -900.378445139689;-0.0019975 -6.73512599400668e-08 -7.68013304391611 -900.377013464181;-0.001997 -6.73512598646342e-08 -7.84984997512892 -900.37554979776;-0.0019965 -6.7351259789202e-08 -8.01956662743204 -900.374054140477;-0.001996 -6.73512597137702e-08 -8.18928299479543 -900.372526492386;-0.0019955 -6.73512596383389e-08 -8.35899907118859 -900.37096685354;-0.001995 -6.73512595629081e-08 -8.52871485058202 -900.369375223996;-0.0019945 -6.73512594874778e-08 -8.69843032694516 -900.367751603809;-0.001994 -6.7351259412048e-08 -8.8681454942481 -900.366095993037;-0.0019935 -6.73512593366186e-08 -9.0378603464608 -900.36440839174;-0.001993 -6.73512592611897e-08 -9.20757487755302 -900.362688799977;-0.0019925 -6.73512591857613e-08 -9.37728908149479 -900.36093721781;-0.001992 -6.73512591103334e-08 -9.54700295225594 -900.3591536453;-0.0019915 -6.7351259034906e-08 -9.7167164838068 -900.35733808251;-0.001991 -6.7351258959479e-08 -9.88642967011711 -900.355490529507;-0.0019905 -6.73512588840526e-08 -10.0561425051569 -900.353610986354;-0.00199 -6.73512588086266e-08 -10.2258549828962 -900.351699453119;-0.0019895 -6.73512587332012e-08 -10.3955670973049 -900.34975592987;-0.001989 -6.73512586577763e-08 -10.5652788423528 -900.347780416675;-0.0019885 -6.73512585823518e-08 -10.7349902120106 -900.345772913606;-0.001988 -6.73512585069279e-08 -10.904701200248 -900.343733420733;-0.0019875 -6.73512584315045e-08 -11.0744118010351 -900.341661938129;-0.001987 -6.73512583560816e-08 -11.244122008342 -900.339558465867;-0.0019865 -6.73512582806592e-08 -11.4138318161387 -900.337423004022;-0.001986 -6.73512582052373e-08 -11.5835412183955 -900.33525555267;-0.0019855 -6.7351258129816e-08 -11.7532502090822 -900.333056111889;-0.001985 -6.73512580543952e-08 -11.9229587821692 -900.330824681755;-0.0019845 -6.73512579789749e-08 -12.0926669316267 -900.328561262349;-0.001984 -6.73512579035551e-08 -12.2623746514248 -900.326265853751;-0.0019835 -6.73512578281359e-08 -12.4320819355336 -900.323938456042;-0.001983 -6.73512577527172e-08 -12.6017887779234 -900.321579069305;-0.0019825 -6.73512576772991e-08 -12.7714951725643 -900.319187693624;-0.001982 -6.73512576018814e-08 -12.9412011134268 -900.316764329085;-0.0019815 -6.73512575264644e-08 -13.1109065944809 -900.314308975772;-0.001981 -6.73512574510478e-08 -13.2806116096969 -900.311821633773;-0.0019805 -6.73512573756319e-08 -13.4503161530451 -900.309302303177;-0.00198 -6.73512573002165e-08 -13.6200202184959 -900.306750984073;-0.0019795 -6.73512572248016e-08 -13.7897238000196 -900.304167676552;-0.001979 -6.73512571493873e-08 -13.9594268915862 -900.301552380706;-0.0019785 -6.73512570739735e-08 -14.1291294871666 -900.298905096627;-0.001978 -6.73512569985603e-08 -14.2988315807308 -900.29622582441;-0.0019775 -6.73512569231477e-08 -14.4685331662493 -900.293514564149;-0.001977 -6.73512568477356e-08 -14.6382342376925 -900.290771315942;-0.0019765 -6.73512567723241e-08 -14.8079347890308 -900.287996079885;-0.001976 -6.73512566969132e-08 -14.9776348142345 -900.285188856077;-0.0019755 -6.73512566215029e-08 -15.1473343072744 -900.282349644618;-0.001975 -6.73512565460931e-08 -15.3170332621207 -900.279478445609;-0.0019745 -6.73512564706839e-08 -15.486731672744 -900.276575259152;-0.001974 -6.73512563952753e-08 -15.6564295331149 -900.273640085349;-0.0019735 -6.73512563198673e-08 -15.8261268372037 -900.270672924306;-0.001973 -6.73512562444599e-08 -15.9958235789813 -900.267673776128;-0.0019725 -6.73512561690531e-08 -16.1655197524178 -900.264642640921;-0.001972 -6.73512560936468e-08 -16.3352153514843 -900.261579518793;-0.0019715 -6.73512560182412e-08 -16.5049103701511 ...(+268233 chars)]  x5=0.002  V1=[7.133e-10 1.392e+04 1.392e+04;377 377 377;1.676 0.5123 -1.059]  V2=[7.264e-10 1.392e+04 1.392e+04;377 377 377;1.669 0.5123 -1.059]  I1=[1.636e-12 51.4 51.4;377 377 377;0.6309 0.5058 -1.065]  I2=[1.868e-12 51.4 51.4;377 377 377;2.957 0.5123 -1.059]  nHarmo=1  Measurements=None
      settings: SourceProductName=Simscape Electrical
  50w load : powerlib/Elements/Three-Phase Series RLC Load  LConnTagsString=A|B|C  Configuration=Y (grounded)  NominalVoltage=220e3  Vabc=[1e3 1e3 1e3]  Vabcp=[1e3 1e3 1e3]  NominalFrequency=50  UnbalancedPower=off  ActivePower=50  InductivePower=0  CapacitivePower=0  Pabc=[10e3 9e3 11e3]  QLabc=[100 90 110]  QCabc=[100 90 110]  Pabcp=[10e3 9e3 11e3]  QLabcp=[100 90 110]  QCabcp=[100 90 110]  Measurements=None  LoadType=constant Z
      settings: SourceProductName=Simscape Electrical
  70w load : powerlib/Elements/Three-Phase Series RLC Load  LConnTagsString=A|B|C  Configuration=Y (grounded)  NominalVoltage=220e3  Vabc=[1e3 1e3 1e3]  Vabcp=[1e3 1e3 1e3]  NominalFrequency=50  UnbalancedPower=off  ActivePower=70  InductivePower=0  CapacitivePower=0  Pabc=[10e3 9e3 11e3]  QLabc=[100 90 110]  QCabc=[100 90 110]  Pabcp=[10e3 9e3 11e3]  QLabcp=[100 90 110]  QCabcp=[100 90 110]  Measurements=None  LoadType=constant Z
      settings: SourceProductName=Simscape Electrical
  Add : Sum  Inputs=+-
  Add{1..6} (6 alike) : Sum  Commented=on  Inputs=+-
  Bus Selector : BusSelector  OutputSignals=Rotor speed wm (rad/s)
  Compare To Zero{,1..5} (6 alike) : simulink/Logic and Bit Operations/Compare To Zero  Commented=on  relop=>=  OutDataTypeStr=boolean
  Constant : Constant  Value=300
  Constant1 : Constant  Value=0
  Current Measurement : powerlib/Measurements/Current Measurement  PhasorSimulation=off  OutputType=Complex  PSBequivalent=0
      settings: SourceProductName=Simscape Electrical
  DC Voltage Source : powerlib/Electrical Sources/DC Voltage Source  Amplitude=-140  Measurements=None
      settings: SourceProductName=Simscape Electrical
  DC Voltage Source1 : powerlib/Electrical Sources/DC Voltage Source  Amplitude=-140  Measurements=None
      settings: SourceProductName=Simscape Electrical
  DC Voltage Source2 : powerlib/Electrical Sources/DC Voltage Source  Amplitude=-140  Measurements=None
      settings: SourceProductName=Simscape Electrical
  Demux : Demux  Outputs=3
  Diode1 : powerlib/Power Electronics/Diode  Ron=0.001  Lon=0  Vf=0.8  IC=0  UseSnubber=0  Rs=500  Cs=250e-9  Measurements=off
      settings: SourceProductName=Simscape Electrical
  From3 : From  Commented=on  GotoTag=S2
  From9 : From  Commented=on  GotoTag=switch2
  Goto : Goto  Commented=on  GotoTag=S1
  Goto1 : Goto  Commented=on  GotoTag=S2
  Goto10 : Goto  Commented=on  GotoTag=switch5
  Goto11 : Goto  Commented=on  GotoTag=switch6
  Goto2 : Goto  Commented=on  GotoTag=S3
  Goto3 : Goto  Commented=on  GotoTag=S4
  Goto4 : Goto  Commented=on  GotoTag=S5
  Goto5 : Goto  Commented=on  GotoTag=S6
  Goto6 : Goto  Commented=on  GotoTag=switch1
  Goto7 : Goto  Commented=on  GotoTag=switch2
  Goto8 : Goto  Commented=on  GotoTag=switch3
  Goto9 : Goto  Commented=on  GotoTag=switch4
  Ground : powerlib/Elements/Ground  LConnTagsString=a
      settings: SourceProductName=Simscape Electrical
  Ground1 : powerlib/Elements/Ground  LConnTagsString=a
      settings: SourceProductName=Simscape Electrical
  "L filter " : powerlib/Elements/Three-Phase Series RLC Branch  LConnTagsString=A|B|C  RConnTagsString=A|B|C  BranchType=L  Resistance=1  Inductance=21.86  Capacitance=1e-6  Measurements=None
      settings: SourceProductName=Simscape Electrical
  Logical Operator{,1..5} (6 alike) : Logic  Commented=on  Operator=NOT  AllPortsSameDT=off  OutDataTypeStr=boolean
  Mosfet{,3..6,9..12} (9 alike) : powerlib/Power Electronics/Mosfet  Ron=0.1  Lon=0  Rd=0.01  Vfd=0  IC=0  Rs=1e5  Cs=inf  Measurements=off
      settings: SourceProductName=Simscape Electrical
  Mosfet{1..2,7..8} (4 alike) : powerlib/Power Electronics/Mosfet  Commented=on  Ron=0.1  Lon=0  Rd=0.01  Vfd=0  IC=0  Rs=1e5  Cs=inf  Measurements=off
      settings: SourceProductName=Simscape Electrical
  Permanent Magnet Synchronous Machine : powerlib/Machines/Permanent Magnet Synchronous Machine  NbPhases=3  FluxDistribution=Sinusoidal  RotorType=Round  MechanicalLoad=Torque Tm  PresetModel="16:  111 Nm 560 Vdc 3000 RPM - 126 Nm"  ShowDetailedParameters=on  MeasurementBus=off  Resistance=0.05  Inductance=8.5e-3  dqInductances=[0.0007932 0.0008767]  La=0.000635  MachineConstant=Flux linkage established by magnets (V.s)  Flux=0.192  VoltageCst=139.2998  TorqueCst=1.152  Flat=120  Mechanical=[0.011 0.001889 4 0]  PolePairs=4  InitialConditions=[0,0, 0,0]  InitialConditions5ph=[0 0 0 0 0 0]  TsPowergui=0  TsBlock=-1  RefAngle=90 degrees behind phase A axis (modified Park)
  Product : Product
  RMS : dspstat3/RMS  run=off  directionMode=Each column  dimension=1  InputProcessing=Columns as channels (frame based)  reset_popup=None
  RMS1 : dspstat3/RMS  run=off  directionMode=Each column  dimension=1  InputProcessing=Columns as channels (frame based)  reset_popup=None
  Relational Operator : RelationalOperator  OutDataTypeStr=boolean  RndMeth=Simplest
  Repeating Sequence : simulink/Sources/Repeating Sequence  rep_seq_t=[0 0.00004]  rep_seq_y=[0 1]
  Repeating Sequence1 : simulink/Sources/Repeating Sequence  Commented=on  rep_seq_t=[0 .5 1]/6750  rep_seq_y=[-1 1 -1]
  Repeating Sequence2 : simulink/Sources/Repeating Sequence  Commented=on  rep_seq_t=[0 .5 1]/6750  rep_seq_y=[-1 1 -1]
  Saturation : Saturate  UpperLimit=.1  LowerLimit=0
  Scope{,1..6,9} (8 alike) : Scope
  Scope7 : Scope  NumInputPorts=3
  Series RLC Branch : powerlib/Elements/Series RLC Branch  LConnTagsString=__new0  RConnTagsString=__new0  BranchType=C  Resistance=1  Inductance=1e-3  SetiL0=off  InitialCurrent=0  Capacitance=1e-1  Setx0=off  InitialVoltage=0  Measurements=None
      settings: SourceProductName=Simscape Electrical
  Series RLC Branch1 : powerlib/Elements/Series RLC Branch  LConnTagsString=__new0  RConnTagsString=__new0  BranchType=R  Resistance=25  Inductance=1e-3  SetiL0=off  InitialCurrent=0  Capacitance=1e-6  Setx0=off  InitialVoltage=0  Measurements=None
      settings: SourceProductName=Simscape Electrical
  Series RLC Branch2 : powerlib/Elements/Series RLC Branch  LConnTagsString=__new0  RConnTagsString=__new0  BranchType=C  Resistance=1  Inductance=1e-3  SetiL0=off  InitialCurrent=0  Capacitance=.25e-2  Setx0=off  InitialVoltage=0  Measurements=None
      settings: SourceProductName=Simscape Electrical
  Series RLC Branch3 : powerlib/Elements/Series RLC Branch  LConnTagsString=__new0  RConnTagsString=__new0  BranchType=L  Resistance=1  Inductance=2.13e-3  SetiL0=off  InitialCurrent=0  Capacitance=1e-6  Setx0=off  InitialVoltage=0  Measurements=None
      settings: SourceProductName=Simscape Electrical
  Series RLC Branch4 : powerlib/Elements/Series RLC Branch  LConnTagsString=__new0  RConnTagsString=__new0  BranchType=R  Resistance=1  Inductance=1e-3  SetiL0=off  InitialCurrent=0  Capacitance=1e-6  Setx0=off  InitialVoltage=0  Measurements=None
      settings: SourceProductName=Simscape Electrical
  Signal Builder : Subsystem  Tag=STV Subsys  LoadFcn=sigbuilder_block('load');  StartFcn=sigbuilder_block('start');  StopFcn=sigbuilder_block('stop');  ClipboardFcn=sigbuilder_block('clipboard');  mask(Sigbuilder block){tuvar=[0:10]}
      mask help: Simulink:masks:SigbuilderBlock_MD
      mask init:
      | if ~strcmp(get_param(bdroot(gcbh),'SimulationStatus'),'stopped') tuvar = sigbuilder_block('maskInit'); end
      settings: CopyFcn=sigbuilder_block('copy');  DeleteFcn=sigbuilder_block('delete');  ModelCloseFcn=sigbuilder_block('modelClose');  PreSaveFcn=sigbuilder_block('preSave');  PauseFcn=sigbuilder_block('pause');  ContinueFcn=sigbuilder_block('continue');  NameChangeFcn=sigbuilder_block('namechange');  OpenFcn=sigbuilder_block('open',[6 30 1012.5 482.25 ]);  CloseFcn=sigbuilder_block('close');
      mask Display: plot(0, 0, 100, 100,[2, 2, 32, 32, 2], [68, 8, 8, 68, 68],[32, 2], [38, 38], [32, 19, 2],[53, 60, 44], [32, 17, 17, 2],[16, 16, 31, 31]);txt = getActiveGroup(gcbh);text(2, 100, txt,'verticalAlignment', 'top');
  Sine Wave : Sin  Commented=on  Amplitude=.8  Frequency=2*pi*50  SampleTime=0
  Sine Wave1 : Sin  Commented=on  Amplitude=.8  Frequency=2*pi*50  Phase=-(2*pi)/3  SampleTime=0
  Sine Wave2 : Sin  Commented=on  Amplitude=.8  Frequency=2*pi*50  Phase=(2*pi)/3  SampleTime=0
  Sine Wave3 : Sin  Commented=on  Amplitude=.8  Frequency=2*pi*50  SampleTime=0
  Sine Wave4 : Sin  Commented=on  Amplitude=.8  Frequency=2*pi*50  Phase=-(2*pi)/3  SampleTime=0
  Sine Wave5 : Sin  Commented=on  Amplitude=.8  Frequency=2*pi*50  Phase=(2*pi)/3  SampleTime=0
  Three-Phase Series RLC Branch : powerlib/Elements/Three-Phase Series RLC Branch  LConnTagsString=A|B|C  RConnTagsString=A|B|C  BranchType=R  Resistance=1  Inductance=1e-3  Capacitance=1e-6  Measurements=None
      settings: SourceProductName=Simscape Electrical
  Three-Phase Series RLC Branch2 : powerlib/Elements/Three-Phase Series RLC Branch  LConnTagsString=A|B|C  RConnTagsString=A|B|C  BranchType=C  Resistance=1  Inductance=1e-3  Capacitance=.1e-6  Measurements=None
      settings: SourceProductName=Simscape Electrical
  Three-Phase Transformer (Two Windings)1 : powerlib/Elements/Three-Phase Transformer (Two Windings)  Winding1Connection=Yg  Winding2Connection=Yg  CoreType=Three single-phase transformers  SetSaturation=off  Hysteresis=off  DataFile='hysteresis'  SetInitialFlux=off  Measurements=None  UNITS=SI  NominalPower=[ sqrt(3)*100 , 50 ]  Winding1=[11e3*sqrt(1/2) 0 0]  Winding2=[220e3*sqrt(1/2) 0 0]  Rm=Inf  Lm=Inf  L0=0.5  Saturation=[0 0;0.83728 285.89;348.87 362.13]  InitialFluxes=[190.59 -190.59 166.77]  BreakLoop=off  DiscreteSolver=Trapezoidal iterative  DataType=on  TransfoNumber=1
      settings: SourceProductName=Simscape Electrical
  Three-Phase Transformer (Two Windings)2 : powerlib/Elements/Three-Phase Transformer (Two Windings)  Winding1Connection=Yg  Winding2Connection=Yg  CoreType=Three single-phase transformers  SetSaturation=off  Hysteresis=off  DataFile='hysteresis'  SetInitialFlux=off  Measurements=None  UNITS=SI  NominalPower=[ sqrt(3)*100 , 50 ]  Winding1=[150*sqrt(1/2) 0 0]  Winding2=[220e3*sqrt(1/2) 0 0]  Rm=Inf  Lm=Inf  L0=0.5  Saturation=[0 0;0.83728 285.89;348.87 362.13]  InitialFluxes=[190.59 -190.59 166.77]  BreakLoop=off  DiscreteSolver=Trapezoidal iterative  DataType=on  TransfoNumber=1
      settings: SourceProductName=Simscape Electrical
  Three-Phase Transformer (Two Windings)3 : powerlib/Elements/Three-Phase Transformer (Two Windings)  Winding1Connection=Yg  Winding2Connection=Yg  CoreType=Three single-phase transformers  SetSaturation=off  Hysteresis=off  DataFile='hysteresis'  SetInitialFlux=off  Measurements=None  UNITS=SI  NominalPower=[ sqrt(3)*100 ,50 ]  Winding1=[11e3*sqrt(1/2) 0 0]  Winding2=[220e3*sqrt(1/2) 0 0]  Rm=Inf  Lm=Inf  L0=0.5  Saturation=[0 0;0.83728 285.89;348.87 362.13]  InitialFluxes=[190.59 -190.59 166.77]  BreakLoop=off  DiscreteSolver=Trapezoidal iterative  DataType=on  TransfoNumber=1
      settings: SourceProductName=Simscape Electrical
  Three-Phase V-I Measurement : powerlib/Measurements/Three-Phase V-I Measurement  VoltageMeasurement=phase-to-ground  SetLabelV=off  LabelV=Vabc  Vpu=off  VpuLL=off  CurrentMeasurement=yes  SetLabelI=off  LabelI=Iabc  Ipu=off  Pbase=100e6  Vbase=500e3  OutputType=Complex  PhasorSimulation=off  PSBequivalent=0
      settings: SourceProductName=Simscape Electrical
  Three-Phase V-I Measurement1 : powerlib/Measurements/Three-Phase V-I Measurement  VoltageMeasurement=phase-to-ground  SetLabelV=off  LabelV=Vabc  Vpu=off  VpuLL=off  CurrentMeasurement=yes  SetLabelI=off  LabelI=Iabc  Ipu=off  Pbase=100e6  Vbase=500e3  OutputType=Complex  PhasorSimulation=off  PSBequivalent=0
      settings: SourceProductName=Simscape Electrical
  Three-Phase V-I Measurement2 : powerlib/Measurements/Three-Phase V-I Measurement  VoltageMeasurement=phase-to-ground  SetLabelV=off  LabelV=Vabc  Vpu=off  VpuLL=off  CurrentMeasurement=no  SetLabelI=off  LabelI=Iabc  Ipu=off  Pbase=100e6  Vbase=500e3  OutputType=Complex  PhasorSimulation=off  PSBequivalent=0
      settings: SourceProductName=Simscape Electrical
  Universal Bridge : powerlib/Power Electronics/Universal Bridge  Arms=3  SnubberResistance=1e5  SnubberCapacitance=inf  Device=Diodes  Ron=1e-3  Lon=0  ForwardVoltages="[  0  0  ]"  ForwardVoltage=0  GTOparameters=[ 10e-6 , 20e-6 ]  IGBTparameters=[ 1e-6 , 2e-6 ]  Measurements=None  Measurements_2=None  converterType=Rectifier
      settings: SourceProductName=Simscape Electrical
  Voltage Measurement : powerlib/Measurements/Voltage Measurement  PhasorSimulation=off  OutputType=Complex  PSBequivalent=0
      settings: SourceProductName=Simscape Electrical
  Voltage Measurement1 : powerlib/Measurements/Voltage Measurement  PhasorSimulation=off  OutputType=Complex  PSBequivalent=0
      settings: SourceProductName=Simscape Electrical
  Wind Turbine : re_lib/Wind Generation/Wind Turbine  Pnom=1.5e6  Pelec_base=1.5e6/0.9  wind_base=0.1  P_wind_base=0.75  speed_nom=0.8  pitch_angle=10  c1_c6="[0.51763          116          0.4            5           21     0.006795]"  cp_nom=0.48  lambda_nom=8.1
      settings: SourceProductName=Simscape Electrical  SourceProductBaseCode=PS
  Zener Diode : Subsystem  mask(Zener Diode){Vz=30, Rzt=10, Rzk=400, Izm=400e-3, Vf=0.7, Ron=1e-3}
      mask prompts: Vz "Zener Voltage Vz (V)"; Rzt "Dynamic Impedance Zzt (ohms)"; Rzk "Knee Impedance Zzk (ohms)"; Izm "Maximum Continuous Current Izm (A)"; Vf "Forward Voltage Drop Vf (V)"; Ron "On Resistance Ron (ohms)"
      mask help:
      | Implements a zener diode block.
      | Use values from standard datasheets to populate block dialog
  powergui : powerlib/powergui  Priority=1  SimulationMode=Discrete  SampleTime=.5e-6  frequency=60  Iterations=50  frequencyindice=0  Pbase=100e6  ErrMax=1e-4  UnitsV=kV  UnitsW=MW  buscounter=0  FunctionMessages=off  echomessages=off  EnableUseOfTLC=off  CurrentSourceSwitches=off  DisableSnubberDevices=off  DisableRonSwitches=off  DisableVfSwitches=off  DisplayEquations=off  AutomaticDiscreteSolvers=off  SolverType=Tustin/Backward Euler (TBE)  Interpol=off  ExternalGateDelay=off  methode=off  Ts=100  x0status=blocks  SPID=on  SwTol=0  HookPort=off  NonlinearTolerance=0  nMaxIteration=15  ContinueOnMaxIteration=off  RestoreLinks=warning  ResistiveCurrentMeasurement=off  Frange=[0:2:500]  Ylog=off  Xlog=on  ShowGrid=off  save=off  variable=ZData  structure=0  ZoomFFT=off  StartTime=0.0  cycles=1  DisplayStyle=1  fundamental=60  FreqAxis=off  MaxFrequency=1000  frequencyindicesteady=1  RmsSteady=1  display=off
      settings: SourceProductName=Simscape Electrical
  wires:
  Demux/1 -> Scope7/1
  Three-Phase V-I Measurement/1 -> RMS/1, Scope3/1
  Three-Phase V-I Measurement2/1 -> Demux/1
  Demux/3 -> Scope7/3
  Voltage Measurement/1 -> Scope5/1
  Add/1 -> Saturation/1
  Demux/2 -> Scope7/2
  Voltage Measurement1/1 -> Scope1/1, Add/2
  Repeating Sequence/1 -> Relational Operator/1
  Signal Builder/1(Signal 1) -> Wind Turbine/3
  Relational Operator/1 -> Mosfet/1
  Permanent Magnet Synchronous Machine/1 -> Bus Selector/1
  Constant/1 -> Add/1
  Saturation/1 -> Relational Operator/2
  Bus Selector/1 -> Scope2/1, Wind Turbine/1  "<Rotor speed wm (rad/s)>"
  Wind Turbine/1 -> Permanent Magnet Synchronous Machine/1, Scope/1
  Three-Phase V-I Measurement1/1 -> Scope6/1
  Constant1/1 -> Wind Turbine/2
  Current Measurement/1 -> Scope4/1
  RMS1/1 -> Product/2
  Product/1 -> Scope9/1
  Three-Phase V-I Measurement/2 -> RMS1/1
  RMS/1 -> Product/1
  Logical Operator/1 -> Goto1/1
  Compare To Zero/1 -> Logical Operator/1, Goto/1
  Sine Wave1/1 -> Add2/1
  Sine Wave2/1 -> Add3/1
  Add1/1 -> Compare To Zero/1
  [S6] -> Mosfet6/1
  [S5] -> Mosfet5/1
  Sine Wave/1 -> Add1/1
  Logical Operator1/1 -> Goto3/1
  Add2/1 -> Compare To Zero1/1
  Compare To Zero1/1 -> Logical Operator1/1, Goto2/1
  From3/1 -> Mosfet2/1
  Add3/1 -> Compare To Zero3/1
  [S4] -> Mosfet4/1
  Compare To Zero3/1 -> Logical Operator2/1, Goto4/1
  [S1] -> Mosfet1/1
  [S3] -> Mosfet3/1
  Logical Operator2/1 -> Goto5/1
  Repeating Sequence1/1 -> Add1/2, Add2/2, Add3/2
  Logical Operator3/1 -> Goto7/1
  Compare To Zero2/1 -> Logical Operator3/1, Goto6/1
  Sine Wave4/1 -> Add5/1
  Sine Wave5/1 -> Add6/1
  Add4/1 -> Compare To Zero2/1
  [switch6] -> Mosfet12/1
  [switch5] -> Mosfet11/1
  Sine Wave3/1 -> Add4/1
  Logical Operator4/1 -> Goto9/1
  Add5/1 -> Compare To Zero4/1
  Compare To Zero4/1 -> Logical Operator4/1, Goto8/1
  From9/1 -> Mosfet8/1
  Add6/1 -> Compare To Zero5/1
  [switch4] -> Mosfet10/1
  Compare To Zero5/1 -> Logical Operator5/1, Goto10/1
  [switch1] -> Mosfet7/1
  [switch3] -> Mosfet9/1
  Logical Operator5/1 -> Goto11/1
  Repeating Sequence2/1 -> Add4/2, Add5/2, Add6/2
  connections:
  Three-Phase V-I Measurement/LConn2 -- Permanent Magnet Synchronous Machine/LConn2
  Permanent Magnet Synchronous Machine/LConn1 -- Three-Phase V-I Measurement/LConn1
  Permanent Magnet Synchronous Machine/LConn3 -- Three-Phase V-I Measurement/LConn3
  Three-Phase Series RLC Branch/RConn2 -- Three-Phase Series RLC Branch/RConn3 -- Ground/LConn1 -- Three-Phase Series RLC Branch/RConn1
  Mosfet7/LConn1 -- Series RLC Branch1/LConn1 -- Series RLC Branch2/LConn1 -- Diode1/RConn1 -- Voltage Measurement1/LConn1 -- Mosfet11/LConn1 -- Mosfet9/LConn1
  Universal Bridge/RConn1 -- Series RLC Branch3/LConn1 -- Voltage Measurement/LConn1 -- Series RLC Branch4/LConn1 -- Zener Diode/LConn1 -- Series RLC Branch/LConn1
  Mosfet/LConn1 -- Diode1/LConn1 -- Current Measurement/RConn1
  Series RLC Branch3/RConn1 -- Current Measurement/LConn1
  "L filter "/LConn1 -- Three-Phase V-I Measurement1/RConn1
  "L filter "/LConn2 -- Three-Phase V-I Measurement1/RConn2
  Mosfet7/RConn1 -- Three-Phase V-I Measurement1/LConn1 -- Mosfet8/LConn1
  "L filter "/LConn3 -- Three-Phase V-I Measurement1/RConn3
  Mosfet9/RConn1 -- Three-Phase V-I Measurement1/LConn2 -- Mosfet10/LConn1
  Mosfet1/LConn1 -- Mosfet5/LConn1 -- Mosfet3/LConn1
  Mosfet8/RConn1 -- Universal Bridge/RConn2 -- Series RLC Branch/RConn1 -- Zener Diode/RConn1 -- Series RLC Branch4/RConn1 -- Voltage Measurement/LConn2 -- Mosfet/RConn1 -- Series RLC Branch2/RConn1 -- Series RLC Branch1/RConn1 -- Voltage Measurement1/LConn2 -- Mosfet10/RConn1 -- Mosfet12/RConn1
  Mosfet1/RConn1 -- Mosfet2/LConn1
  Mosfet5/RConn1 -- Mosfet6/LConn1
  Mosfet3/RConn1 -- Mosfet4/LConn1
  Mosfet11/RConn1 -- Three-Phase V-I Measurement1/LConn3 -- Mosfet12/LConn1
  Mosfet6/RConn1 -- Mosfet2/RConn1 -- Mosfet4/RConn1
  Three-Phase Series RLC Branch2/LConn1 -- DC Voltage Source/LConn1 -- "L filter "/RConn1
  Three-Phase Series RLC Branch2/LConn2 -- "L filter "/RConn2 -- DC Voltage Source1/LConn1
  Three-Phase Series RLC Branch2/LConn3 -- DC Voltage Source2/LConn1 -- "L filter "/RConn3
  Three-Phase Series RLC Branch2/RConn1 -- Three-Phase Series RLC Branch2/RConn2 -- Ground1/LConn1 -- Three-Phase Series RLC Branch2/RConn3
  DC Voltage Source/RConn1 -- Three-Phase V-I Measurement2/LConn1
  DC Voltage Source1/RConn1 -- Three-Phase V-I Measurement2/LConn2
  DC Voltage Source2/RConn1 -- Three-Phase V-I Measurement2/LConn3
  Three-Phase Transformer (Two Windings)2/LConn2 -- Three-Phase V-I Measurement2/RConn2
  14 km feeder 1/LConn1 -- Three-Phase Transformer (Two Windings)1/LConn1 -- 40w load/LConn1
  50w load/LConn1 -- Three-Phase Transformer (Two Windings)3/RConn1 -- 5 km feeder2/RConn3
  5 km feeder2/LConn3 -- 5 km feeder1/LConn1 -- 70w load/LConn1 -- 14 km feeder 1/RConn1
  14 km feeder 1/RConn2 -- 5 km feeder1/LConn2 -- 70w load/LConn2 -- 5 km feeder2/LConn2
  5 km feeder2/RConn1 -- Three-Phase Transformer (Two Windings)3/RConn3 -- 50w load/LConn3
  14 km feeder 1/RConn3 -- 5 km feeder1/LConn3 -- 70w load/LConn3 -- 5 km feeder2/LConn1
  50w load/LConn2 -- Three-Phase Transformer (Two Windings)3/RConn2 -- 5 km feeder2/RConn2
  Three-Phase Transformer (Two Windings)3/LConn2 -- 11kV source 2/RConn2
  14 km feeder 1/LConn2 -- 40w load/LConn2 -- Three-Phase Transformer (Two Windings)1/LConn2
  Three-Phase Transformer (Two Windings)3/LConn1 -- 11kV source 2/RConn1
  14 km feeder 1/LConn3 -- 40w load/LConn3 -- Three-Phase Transformer (Two Windings)1/LConn3
  Three-Phase Transformer (Two Windings)3/LConn3 -- 11kV source 2/RConn3
  Three-Phase V-I Measurement2/RConn1 -- Three-Phase Transformer (Two Windings)2/LConn1
  Three-Phase Transformer (Two Windings)2/LConn3 -- Three-Phase V-I Measurement2/RConn3
  Three-Phase Transformer (Two Windings)2/RConn1 -- 5 km feeder1/RConn1
  5 km feeder1/RConn2 -- Three-Phase Transformer (Two Windings)2/RConn2
  Three-Phase Transformer (Two Windings)2/RConn3 -- 5 km feeder1/RConn3
  Three-Phase Transformer (Two Windings)1/RConn1 -- 11kV source 1/RConn1
  Three-Phase Transformer (Two Windings)1/RConn2 -- 11kV source 1/RConn2
  11kV source 1/RConn3 -- Three-Phase Transformer (Two Windings)1/RConn3
  Three-Phase V-I Measurement/RConn1 -- Universal Bridge/LConn1 -- Three-Phase Series RLC Branch/LConn1
  Three-Phase V-I Measurement/RConn2 -- Universal Bridge/LConn2 -- Three-Phase Series RLC Branch/LConn2
  Three-Phase V-I Measurement/RConn3 -- Universal Bridge/LConn3 -- Three-Phase Series RLC Branch/LConn3
